simulink model "T6_changeloadmodeltocurrentload_v1"  (R2022b)
settings: Solver=FixedStepAuto  StartTime=0.0  StopTime=48*4  FixedStep=0.01  RelTol=1e-3
undefined symbols (not defined in the file): cableLV, cableMV, High, Low, LV, MV, Scaling_factor, Ts
libraries: fl_lib x149, nesl_utility x73, simulink x60, ee_lib x9
(part 3 of 3)

== system T6_changeloadmodeltocurrentload_v1/Line21 ==
  Current Sensor : fl_lib/Electrical/Electrical Sensors/Current Sensor
  PS-Simulink Converter : nesl_utility/PS-Simulink Converter  PhysicalDomain=network_engine_domain  SubClassName=ps_output  LeftPortType=input  RightPortType=output  PseudoPeriodic=off  Frequencies=[]  VectorFormat=inherit  Unit=inherit  AffineConversion=off
  Resistor : fl_lib/Electrical/Electrical Elements/Resistor  R=rho*l/A Ohm  i_specify=off  i_priority=None  i=0 A  i_nominal_specify=off  i_nominal_unit=A  i_nominal_value=1  v_specify=off  v_priority=None  v=0 V  v_nominal_specify=off  v_nominal_unit=V  v_nominal_value=1
  Resistor1 : fl_lib/Electrical/Electrical Elements/Resistor  R=rho*l/A Ohm  i_specify=off  i_priority=None  i=0 A  i_nominal_specify=off  i_nominal_unit=A  i_nominal_value=1  v_specify=off  v_priority=None  v=0 V  v_nominal_specify=off  v_nominal_unit=V  v_nominal_value=1
  Scope : Scope
  Simscape Bus2 : SimscapeBus  HierarchyStrings=High;Low
  Simscape Bus3 : SimscapeBus  HierarchyStrings=High;Low
  In : PMIOPort  Side=Left
  Out : PMIOPort  Port=2  Side=Right
  wires:
  PS-Simulink Converter/1 -> Scope/1
  connections:
  Simscape Bus2/LConn1 -- Resistor/LConn1
  Simscape Bus3/LConn2 -- Resistor1/RConn1
  Simscape Bus2/RConn1 -- In/RConn1
  Resistor1/LConn1 -- Simscape Bus2/LConn2
  Simscape Bus3/RConn1 -- Out/RConn1
  Current Sensor/LConn1 -- Resistor/RConn1
  Current Sensor/RConn2 -- Simscape Bus3/LConn1
  PS-Simulink Converter/LConn1 -- Current Sensor/RConn1

== system T6_changeloadmodeltocurrentload_v1/Line22 ==
  Current Sensor : fl_lib/Electrical/Electrical Sensors/Current Sensor
  PS-Simulink Converter : nesl_utility/PS-Simulink Converter  PhysicalDomain=network_engine_domain  SubClassName=ps_output  LeftPortType=input  RightPortType=output  PseudoPeriodic=off  Frequencies=[]  VectorFormat=inherit  Unit=inherit  AffineConversion=off
  PS-Simulink Converter1 : nesl_utility/PS-Simulink Converter  PhysicalDomain=network_engine_domain  SubClassName=ps_output  LeftPortType=input  RightPortType=output  PseudoPeriodic=off  Frequencies=[]  VectorFormat=inherit  Unit=inherit  AffineConversion=off
  Resistor : fl_lib/Electrical/Electrical Elements/Resistor  R=rho*l/A Ohm  i_specify=off  i_priority=None  i=0 A  i_nominal_specify=off  i_nominal_unit=A  i_nominal_value=1  v_specify=off  v_priority=None  v=0 V  v_nominal_specify=off  v_nominal_unit=V  v_nominal_value=1
  Resistor1 : fl_lib/Electrical/Electrical Elements/Resistor  R=rho*l/A Ohm  i_specify=off  i_priority=None  i=0 A  i_nominal_specify=off  i_nominal_unit=A  i_nominal_value=1  v_specify=off  v_priority=None  v=0 V  v_nominal_specify=off  v_nominal_unit=V  v_nominal_value=1
  Scope : Scope
  Simscape Bus2 : SimscapeBus  HierarchyStrings=High;Low
  Simscape Bus3 : SimscapeBus  HierarchyStrings=High;Low
  Voltage Sensor : fl_lib/Electrical/Electrical Sensors/Voltage Sensor
  In : PMIOPort  Side=Left
  Out : PMIOPort  Port=2  Side=Right
  tag scope: Bus_Current=global, Bus_Voltage=global
  wires:
  PS-Simulink Converter/1 -> [Bus_Voltage]
  PS-Simulink Converter1/1 -> Scope/1, [Bus_Current]
  connections:
  Simscape Bus3/RConn1 -- Out/RConn1
  Resistor1/LConn1 -- Simscape Bus2/LConn2
  Simscape Bus3/LConn1 -- Voltage Sensor/RConn2 -- Resistor/RConn1
  Simscape Bus2/RConn1 -- In/RConn1
  Simscape Bus3/LConn2 -- Resistor1/RConn1
  PS-Simulink Converter/LConn1 -- Voltage Sensor/RConn1
  Current Sensor/RConn2 -- Voltage Sensor/LConn1 -- Resistor/LConn1
  Current Sensor/LConn1 -- Simscape Bus2/LConn1
  PS-Simulink Converter1/LConn1 -- Current Sensor/RConn1

== system T6_changeloadmodeltocurrentload_v1/Line3 ==
  Resistor : fl_lib/Electrical/Electrical Elements/Resistor  R=rho*l/A Ohm  i_specify=off  i_priority=None  i=0 A  i_nominal_specify=off  i_nominal_unit=A  i_nominal_value=1  v_specify=off  v_priority=None  v=0 V  v_nominal_specify=off  v_nominal_unit=V  v_nominal_value=1
  Resistor1 : fl_lib/Electrical/Electrical Elements/Resistor  R=rho*l/A Ohm  i_specify=off  i_priority=None  i=0 A  i_nominal_specify=off  i_nominal_unit=A  i_nominal_value=1  v_specify=off  v_priority=None  v=0 V  v_nominal_specify=off  v_nominal_unit=V  v_nominal_value=1
  Simscape Bus2 : SimscapeBus  HierarchyStrings=High;Low
  Simscape Bus3 : SimscapeBus  HierarchyStrings=High;Low
  In : PMIOPort  Side=Left
  Out : PMIOPort  Port=2  Side=Right
  connections:
  Simscape Bus2/LConn1 -- Resistor/LConn1
  Simscape Bus3/LConn2 -- Resistor1/RConn1
  Simscape Bus2/RConn1 -- In/RConn1
  Simscape Bus3/LConn1 -- Resistor/RConn1
  Resistor1/LConn1 -- Simscape Bus2/LConn2
  Simscape Bus3/RConn1 -- Out/RConn1

== system T6_changeloadmodeltocurrentload_v1/Line4 ==
  Resistor : fl_lib/Electrical/Electrical Elements/Resistor  R=rho*l/A Ohm  i_specify=off  i_priority=None  i=0 A  i_nominal_specify=off  i_nominal_unit=A  i_nominal_value=1  v_specify=off  v_priority=None  v=0 V  v_nominal_specify=off  v_nominal_unit=V  v_nominal_value=1
  Resistor1 : fl_lib/Electrical/Electrical Elements/Resistor  R=rho*l/A Ohm  i_specify=off  i_priority=None  i=0 A  i_nominal_specify=off  i_nominal_unit=A  i_nominal_value=1  v_specify=off  v_priority=None  v=0 V  v_nominal_specify=off  v_nominal_unit=V  v_nominal_value=1
  Simscape Bus2 : SimscapeBus  HierarchyStrings=High;Low
  Simscape Bus3 : SimscapeBus  HierarchyStrings=High;Low
  In : PMIOPort  Side=Left
  Out : PMIOPort  Port=2  Side=Right
  connections:
  Simscape Bus3/RConn1 -- Out/RConn1
  Resistor1/LConn1 -- Simscape Bus2/LConn2
  Simscape Bus3/LConn1 -- Resistor/RConn1
  Simscape Bus2/RConn1 -- In/RConn1
  Simscape Bus3/LConn2 -- Resistor1/RConn1
  Simscape Bus2/LConn1 -- Resistor/LConn1

== system T6_changeloadmodeltocurrentload_v1/Line5 ==
  Resistor : fl_lib/Electrical/Electrical Elements/Resistor  R=rho*l/A Ohm  i_specify=off  i_priority=None  i=0 A  i_nominal_specify=off  i_nominal_unit=A  i_nominal_value=1  v_specify=off  v_priority=None  v=0 V  v_nominal_specify=off  v_nominal_unit=V  v_nominal_value=1
  Resistor1 : fl_lib/Electrical/Electrical Elements/Resistor  R=rho*l/A Ohm  i_specify=off  i_priority=None  i=0 A  i_nominal_specify=off  i_nominal_unit=A  i_nominal_value=1  v_specify=off  v_priority=None  v=0 V  v_nominal_specify=off  v_nominal_unit=V  v_nominal_value=1
  Simscape Bus2 : SimscapeBus  HierarchyStrings=High;Low
  Simscape Bus3 : SimscapeBus  HierarchyStrings=High;Low
  In : PMIOPort  Side=Left
  Out : PMIOPort  Port=2  Side=Right
  connections:
  Simscape Bus2/LConn1 -- Resistor/LConn1
  Simscape Bus3/LConn2 -- Resistor1/RConn1
  Simscape Bus2/RConn1 -- In/RConn1
  Simscape Bus3/LConn1 -- Resistor/RConn1
  Resistor1/LConn1 -- Simscape Bus2/LConn2
  Simscape Bus3/RConn1 -- Out/RConn1

== system T6_changeloadmodeltocurrentload_v1/Line6 ==
  Resistor : fl_lib/Electrical/Electrical Elements/Resistor  R=rho*l/A Ohm  i_specify=off  i_priority=None  i=0 A  i_nominal_specify=off  i_nominal_unit=A  i_nominal_value=1  v_specify=off  v_priority=None  v=0 V  v_nominal_specify=off  v_nominal_unit=V  v_nominal_value=1
  Resistor1 : fl_lib/Electrical/Electrical Elements/Resistor  R=rho*l/A Ohm  i_specify=off  i_priority=None  i=0 A  i_nominal_specify=off  i_nominal_unit=A  i_nominal_value=1  v_specify=off  v_priority=None  v=0 V  v_nominal_specify=off  v_nominal_unit=V  v_nominal_value=1
  Simscape Bus2 : SimscapeBus  HierarchyStrings=High;Low
  Simscape Bus3 : SimscapeBus  HierarchyStrings=High;Low
  In : PMIOPort  Side=Left
  Out : PMIOPort  Port=2  Side=Right
  connections:
  Simscape Bus3/RConn1 -- Out/RConn1
  Resistor1/LConn1 -- Simscape Bus2/LConn2
  Simscape Bus3/LConn1 -- Resistor/RConn1
  Simscape Bus2/RConn1 -- In/RConn1
  Simscape Bus3/LConn2 -- Resistor1/RConn1
  Simscape Bus2/LConn1 -- Resistor/LConn1

== system T6_changeloadmodeltocurrentload_v1/Line7 ==
  Resistor : fl_lib/Electrical/Electrical Elements/Resistor  R=rho*l/A Ohm  i_specify=off  i_priority=None  i=0 A  i_nominal_specify=off  i_nominal_unit=A  i_nominal_value=1  v_specify=off  v_priority=None  v=0 V  v_nominal_specify=off  v_nominal_unit=V  v_nominal_value=1
  Resistor1 : fl_lib/Electrical/Electrical Elements/Resistor  R=rho*l/A Ohm  i_specify=off  i_priority=None  i=0 A  i_nominal_specify=off  i_nominal_unit=A  i_nominal_value=1  v_specify=off  v_priority=None  v=0 V  v_nominal_specify=off  v_nominal_unit=V  v_nominal_value=1
  Simscape Bus2 : SimscapeBus  HierarchyStrings=High;Low
  Simscape Bus3 : SimscapeBus  HierarchyStrings=High;Low
  In : PMIOPort  Side=Left
  Out : PMIOPort  Port=2  Side=Right
  connections:
  Simscape Bus2/LConn1 -- Resistor/LConn1
  Simscape Bus3/LConn2 -- Resistor1/RConn1
  Simscape Bus2/RConn1 -- In/RConn1
  Simscape Bus3/LConn1 -- Resistor/RConn1
  Resistor1/LConn1 -- Simscape Bus2/LConn2
  Simscape Bus3/RConn1 -- Out/RConn1

== system T6_changeloadmodeltocurrentload_v1/Line8 ==
  Current Sensor : fl_lib/Electrical/Electrical Sensors/Current Sensor
  PS-Simulink Converter : nesl_utility/PS-Simulink Converter  PhysicalDomain=network_engine_domain  SubClassName=ps_output  LeftPortType=input  RightPortType=output  PseudoPeriodic=off  Frequencies=[]  VectorFormat=inherit  Unit=inherit  AffineConversion=off
  Resistor : fl_lib/Electrical/Electrical Elements/Resistor  R=rho*l/A Ohm  i_specify=off  i_priority=None  i=0 A  i_nominal_specify=off  i_nominal_unit=A  i_nominal_value=1  v_specify=off  v_priority=None  v=0 V  v_nominal_specify=off  v_nominal_unit=V  v_nominal_value=1
  Resistor1 : fl_lib/Electrical/Electrical Elements/Resistor  R=rho*l/A Ohm  i_specify=off  i_priority=None  i=0 A  i_nominal_specify=off  i_nominal_unit=A  i_nominal_value=1  v_specify=off  v_priority=None  v=0 V  v_nominal_specify=off  v_nominal_unit=V  v_nominal_value=1
  Scope : Scope
  Simscape Bus2 : SimscapeBus  HierarchyStrings=High;Low
  Simscape Bus3 : SimscapeBus  HierarchyStrings=High;Low
  In : PMIOPort  Side=Left
  Out : PMIOPort  Port=2  Side=Right
  wires:
  PS-Simulink Converter/1 -> Scope/1
  connections:
  Simscape Bus2/LConn1 -- Resistor/LConn1
  Simscape Bus3/LConn2 -- Resistor1/RConn1
  Simscape Bus2/RConn1 -- In/RConn1
  Resistor1/LConn1 -- Simscape Bus2/LConn2
  Simscape Bus3/RConn1 -- Out/RConn1
  Resistor/RConn1 -- Current Sensor/LConn1
  Current Sensor/RConn2 -- Simscape Bus3/LConn1
  PS-Simulink Converter/LConn1 -- Current Sensor/RConn1

== system T6_changeloadmodeltocurrentload_v1/Line9 ==
  Resistor : fl_lib/Electrical/Electrical Elements/Resistor  R=rho*l/A Ohm  i_specify=off  i_priority=None  i=0 A  i_nominal_specify=off  i_nominal_unit=A  i_nominal_value=1  v_specify=off  v_priority=None  v=0 V  v_nominal_specify=off  v_nominal_unit=V  v_nominal_value=1
  Resistor1 : fl_lib/Electrical/Electrical Elements/Resistor  R=rho*l/A Ohm  i_specify=off  i_priority=None  i=0 A  i_nominal_specify=off  i_nominal_unit=A  i_nominal_value=1  v_specify=off  v_priority=None  v=0 V  v_nominal_specify=off  v_nominal_unit=V  v_nominal_value=1
  Simscape Bus2 : SimscapeBus  HierarchyStrings=High;Low
  Simscape Bus3 : SimscapeBus  HierarchyStrings=High;Low
  In : PMIOPort  Side=Left
  Out : PMIOPort  Port=2  Side=Right
  connections:
  Simscape Bus3/RConn1 -- Out/RConn1
  Resistor1/LConn1 -- Simscape Bus2/LConn2
  Simscape Bus3/LConn1 -- Resistor/RConn1
  Simscape Bus2/RConn1 -- In/RConn1
  Simscape Bus3/LConn2 -- Resistor1/RConn1
  Simscape Bus2/LConn1 -- Resistor/LConn1

== system T6_changeloadmodeltocurrentload_v1/Solar power ==
  note: -9
  note: -4
  note: Ns series panel
  Irradiance2 : Inport
  Buck/Boost Converter : Subsystem
      settings: PortSchema="{\"entries\":[{\"content\":{\"sides\":[{\"content\":{\"connectorIds\":[\"LConn1\",\"LConn2\"]},\"type\":\"ConnectorPlacement.EquallySpacedRectSide\",\"uuid\":\"5c021c6f-6d43-4834-8d7d-5513bb4d55a2\"},{\"content\":{\"connectorIds\":[\"RConn1\",\"RConn2\"],\"side\":\"RIGHT\"},\"type\":\"ConnectorPlacement.EquallySpacedRectSide\",\"uuid\":\"9a583822-2cc1-49ae-b5aa-706b08d37e90\"},{\"content\":{\"connectorIds\":[\"In1\"],\"side\":\"TOP\"},\"type\":\"ConnectorPlacement.EquallySpacedRectSide\",\"uuid\":\"d4d092e8-f797-44a8-a681-f8c20d4ba78f\"}]},\"type\":\"ConnectorPlacement.EquallySpacedConnector\",\"uuid\":\"2126b667-6bdd-4954-a062-f2cc2f0ec1c9\"}],\"packageUris\":[\"http://schema.mathworks.com/mf0/Connector/R2020b\"],\"version\":\"1.0\"}"
  Current Sensor2 : fl_lib/Electrical/Electrical Sensors/Current Sensor
  Current-Controlled Current Source : fl_lib/Electrical/Electrical Sources/Current-Controlled Current Source  K=-1*(1-1)  i1_specify=off  i1_priority=None  i1=0 A  i1_nominal_specify=off  i1_nominal_unit=A  i1_nominal_value=1  i2_specify=off  i2_priority=None  i2=0 A  i2_nominal_specify=off  i2_nominal_unit=A  i2_nominal_value=1
      settings: InternalSimscapePortConfiguration="{\"Bottom\":[],\"Left\":[{\"id\":\"p1\",\"label\":\"+\",\"type\":\"foundation.electrical.electrical\"},{\"id\":\"head\",\"label\":\"\",\"type\":\"foundation.electrical.electrical\"}],\"Right\":[{\"id\":\"n1\",\"label\":\"-\",\"type\":\"foundation.electrical.electrical\"},{\"id\":\"tail\",\"label\":\"\",\"type\":\"foundation.electrical.electrical\"}],\"Top\":[]}"
  Current-Controlled Current Source- Scale panel current to Np parallel strings : fl_lib/Electrical/Electrical Sources/Current-Controlled Current Source  K=-1*(1-1)  i1_specify=off  i1_priority=None  i1=0 A  i1_nominal_specify=off  i1_nominal_unit=A  i1_nominal_value=1  i2_specify=off  i2_priority=None  i2=0 A  i2_nominal_specify=off  i2_nominal_unit=A  i2_nominal_value=1
      settings: InternalSimscapePortConfiguration="{\"Bottom\":[],\"Left\":[{\"id\":\"p1\",\"label\":\"+\",\"type\":\"foundation.electrical.electrical\"},{\"id\":\"head\",\"label\":\"\",\"type\":\"foundation.electrical.electrical\"}],\"Right\":[{\"id\":\"n1\",\"label\":\"-\",\"type\":\"foundation.electrical.electrical\"},{\"id\":\"tail\",\"label\":\"\",\"type\":\"foundation.electrical.electrical\"}],\"Top\":[]}"
  ERef : fl_lib/Electrical/Electrical Elements/Electrical Reference
  MPPT : Subsystem
  PS-Simulink Converter1 : nesl_utility/PS-Simulink Converter  PhysicalDomain=network_engine_domain  SubClassName=ps_output  LeftPortType=input  RightPortType=output  PseudoPeriodic=off  Frequencies=[]  VectorFormat=1-D array  Unit=inherit  AffineConversion=off
  PS-Simulink Converter4 : nesl_utility/PS-Simulink Converter  PhysicalDomain=network_engine_domain  SubClassName=ps_output  LeftPortType=input  RightPortType=output  PseudoPeriodic=off  Frequencies=[]  VectorFormat=1-D array  Unit=inherit  AffineConversion=off
  Product3 : Product
  Scope : Scope
  Sensing Current : Subsystem
      settings: PortSchema="{\"entries\":[{\"content\":{\"sides\":[{\"content\":{\"connectorIds\":[\"LConn1\"]},\"type\":\"ConnectorPlacement.EquallySpacedRectSide\",\"uuid\":\"08eaf192-3836-4d70-9f6a-c3aee0977ea6\"},{\"content\":{\"connectorIds\":[\"RConn1\"],\"side\":\"RIGHT\"},\"type\":\"ConnectorPlacement.EquallySpacedRectSide\",\"uuid\":\"69615d36-c1bf-4d31-b3e4-77c73286e7c7\"},{\"content\":{\"connectorIds\":[\"Out1\"],\"side\":\"TOP\"},\"type\":\"ConnectorPlacement.EquallySpacedRectSide\",\"uuid\":\"21e31d90-f675-47e5-98f5-1bf7e6a5fdbe\"}]},\"type\":\"ConnectorPlacement.EquallySpacedConnector\",\"uuid\":\"068abd2e-abc9-41d7-b40e-d83d3e3b9346\"}],\"packageUris\":[\"http://schema.mathworks.com/mf0/Connector/R2020b\"],\"version\":\"1.0\"}"
      mask Display: disp('i')
  Simscape Bus1 : SimscapeBus  HierarchyStrings=High;Low
  Simulink-PS Converter2 : nesl_utility/Simulink-PS Converter  PhysicalDomain=network_engine_domain  SubClassName=ps_input  LeftPortType=input  RightPortType=output  PseudoPeriodic=off  Frequencies=[]  NoiseDistribution=none  NoiseParameters=[]  Unit=1  AffineConversion=off  FilteringAndDerivatives=provide  SimscapeFilterOrder=1  InputFilterTimeConstant=0.001  UdotUserProvided=0
  Solar Cell1 : ee_lib/Sources/Solar Cell  Tag={'toolbox/physmod/elec/library/m/ee_lib_parts';'Sources/Solar_Cell/Amerisolar/AS_6M30_HC_320W.xml'}  prm=1  Isc=10.00 A  Voc=0.673 V  Is=3.24823447983853e-07 A  Is2=9.37081970792037e-10 A  Iph=10.140005507508 A  Ir0=1000 W/m^2  ec=1.5  N2=2.60259908345858  Rs=0 Ohm  Rp=682.95993142779 Ohm  N_series=60  N_parallel=1  TIPH1=0.000499942933005141 1/K  EG=1.12 eV  TXIS1=4.23641510120988  TXIS2=16.2689137700667  TRS1=0.243341028305912  TRP1=0 % Parameter not set  Tmeas=25 degC  TFIXED=25 degC  thermal_mass=100 % Parameter not set J/K  initial_temperature=25 degC
      settings: AttributesFormatString=Amerisolar:AS_6M30_HC_320W
  Voltage Sensor2 : fl_lib/Electrical/Electrical Sensors/Voltage Sensor
  Voltage-Controlled Voltage Source - Scale panel voltage to Ns series panel : fl_lib/Electrical/Electrical Sources/Voltage-Controlled Voltage Source  K=-1*(21-1)  v1_specify=off  v1_priority=None  v1=0 V  v1_nominal_specify=off  v1_nominal_unit=V  v1_nominal_value=1  v2_specify=off  v2_priority=None  v2=0 V  v2_nominal_specify=off  v2_nominal_unit=V  v2_nominal_value=1
      settings: InternalSimscapePortConfiguration="{\"Bottom\":[],\"Left\":[{\"id\":\"p1\",\"label\":\"+\",\"type\":\"foundation.electrical.electrical\"},{\"id\":\"p2\",\"label\":\"+\",\"type\":\"foundation.electrical.electrical\"}],\"Right\":[{\"id\":\"n1\",\"label\":\"-\",\"type\":\"foundation.electrical.electrical\"},{\"id\":\"n2\",\"label\":\"-\",\"type\":\"foundation.electrical.electrical\"}],\"Top\":[]}"
  sensing voltage : Subsystem
      settings: PortSchema="{\"entries\":[{\"content\":{\"sides\":[{\"content\":{\"connectorIds\":[\"LConn1\"]},\"type\":\"ConnectorPlacement.EquallySpacedRectSide\",\"uuid\":\"08eaf192-3836-4d70-9f6a-c3aee0977ea6\"},{\"content\":{\"connectorIds\":[\"RConn1\"],\"side\":\"RIGHT\"},\"type\":\"ConnectorPlacement.EquallySpacedRectSide\",\"uuid\":\"69615d36-c1bf-4d31-b3e4-77c73286e7c7\"},{\"content\":{\"connectorIds\":[],\"side\":\"TOP\"},\"type\":\"ConnectorPlacement.EquallySpacedRectSide\",\"uuid\":\"21e31d90-f675-47e5-98f5-1bf7e6a5fdbe\"},{\"content\":{\"connectorIds\":[\"Out1\"],\"side\":\"BOTTOM\"},\"type\":\"ConnectorPlacement.EquallySpacedRectSide\",\"uuid\":\"23a77980-6beb-4147-b48e-adf9e1983263\"}]},\"type\":\"ConnectorPlacement.EquallySpacedConnector\",\"uuid\":\"068abd2e-abc9-41d7-b40e-d83d3e3b9346\"}],\"packageUris\":[\"http://schema.mathworks.com/mf0/Connector/R2020b\"],\"version\":\"1.0\"}"
      mask Display: disp('v')
  solaroutput2 : PMIOPort  Side=Left
  tag scope: MPPT_duty_cycle=global, P_PV=global, V_PV=global, V_PV_load=global
  wires:
  MPPT/1(duty_cycle) -> [MPPT_duty_cycle], Buck/Boost Converter/1(duty_cycle)  "duty_cycle"
  PS-Simulink Converter4/1 -> [V_PV_load], Product3/2  "V_PV_load"
  Sensing Current/1(I) -> MPPT/1(I)
  Irradiance2/1 -> Simulink-PS Converter2/1
  sensing voltage/1(V) -> [V_PV], MPPT/2(V)  "V_cell"
  PS-Simulink Converter1/1 -> Scope/1, Product3/1  "I_PV_load"
  Product3/1 -> [P_PV]  "P_PV"
  connections:
  sensing voltage/RConn1 -- ERef/LConn1 -- Current-Controlled Current Source- Scale panel current to Np parallel strings/LConn2 -- Voltage-Controlled Voltage Source - Scale panel voltage to Ns series panel/LConn1 -- Current-Controlled Current Source/LConn2 -- Solar Cell1/RConn1 -- Buck/Boost Converter/LConn2
  Voltage Sensor2/LConn1 -- Current Sensor2/RConn2 -- Simscape Bus1/LConn1
  Voltage-Controlled Voltage Source - Scale panel voltage to Ns series panel/RConn2 -- Voltage-Controlled Voltage Source - Scale panel voltage to Ns series panel/RConn1 -- Current-Controlled Current Source/RConn1 -- Current-Controlled Current Source/RConn2
  Voltage Sensor2/RConn2 -- Simscape Bus1/LConn2 -- Buck/Boost Converter/RConn2
  Sensing Current/LConn1 -- Current-Controlled Current Source- Scale panel current to Np parallel strings/RConn2 -- Current-Controlled Current Source- Scale panel current to Np parallel strings/RConn1
  Sensing Current/RConn1 -- Buck/Boost Converter/LConn1 -- sensing voltage/LConn1
  solaroutput2/RConn1 -- Simscape Bus1/RConn1
  Solar Cell1/LConn2 -- Current-Controlled Current Source/LConn1
  Buck/Boost Converter/RConn1 -- Current Sensor2/LConn1
  PS-Simulink Converter4/LConn1 -- Voltage Sensor2/RConn1
  Simulink-PS Converter2/RConn1 -- Solar Cell1/LConn1
  Current-Controlled Current Source- Scale panel current to Np parallel strings/LConn1 -- Voltage-Controlled Voltage Source - Scale panel voltage to Ns series panel/LConn2
  PS-Simulink Converter1/LConn1 -- Current Sensor2/RConn1

== system T6_changeloadmodeltocurrentload_v1/Subsystem ==
  "  " : simulink/Sources/Repeating Sequence Interpolated  OutValues=|  TimeValues=Allday_timevector  LookUpMeth=Interpolation-Use End Values  tsamp=0.01  OutMin=[]  OutMax=[]  OutDataTypeStr=double  OutputDataTypeScalingMode=double  OutDataType=fixdt(0,8)  OutScaling=2^-10
      | [2.38
      | 2.43
      | 2.50
      | 2.50
      | 2.45
      | 2.30
      | 2.12
      | 2.15
      | 2.03
      | 2.55
      | 2.97
      | 3.30
      | 3.58
      | 3.83
      | 2.98
      | 2.62
      | 2.53
      | 2.35
      | 2.00
      | 1.72
      | 1.90
      | 2.24
      | 2.15
      | 1.99
      | 1.73
      | 1.40
      | 1.27
      | 1.20
      | 1.43
      | 1.74
      | 1.62
      | 1.35
      | 1.21
      | 1.20
      | 0.98
      | 1.41
      | 1.20
      | 2.08
      | 2.65
      | 2.90
      | 3.03
      | 2.47
      | 2.33
      | 1.97
      | 2.38
      | 3.00
      | 3.01
      | 3.75
      | ]
  "  1" : simulink/Sources/Repeating Sequence Interpolated  OutValues=|  TimeValues=Allday_timevector  LookUpMeth=Interpolation-Use End Values  tsamp=0.01  OutMin=[]  OutMax=[]  OutDataTypeStr=double  OutputDataTypeScalingMode=double  OutDataType=fixdt(0,8)  OutScaling=2^-10
      | [1.52
      | 2.00
      | 2.25
      | 2.19
      | 1.97
      | 1.88
      | 1.99
      | 2.20
      | 2.13
      | 2.47
      | 2.68
      | 2.41
      | 2.85
      | 3.00
      | 3.11
      | 3.38
      | 3.38
      | 3.22
      | 2.93
      | 2.41
      | 1.90
      | 1.46
      | 1.63
      | 1.93
      | 1.93
      | 1.82
      | 1.72
      | 1.76
      | 1.87
      | 2.03
      | 2.21
      | 2.43
      | 2.53
      | 2.73
      | 3.07
      | 2.98
      | 3.38
      | 3.42
      | 3.41
      | 3.57
      | 3.61
      | 3.13
      | 2.60
      | 2.20
      | 1.94
      | 1.79
      | 2.28
      | 2.72
      | ]
  "  2" : simulink/Sources/Repeating Sequence Interpolated  OutValues=|  TimeValues=Allday_timevector  LookUpMeth=Interpolation-Use End Values  tsamp=0.01  OutMin=[]  OutMax=[]  OutDataTypeStr=double  OutputDataTypeScalingMode=double  OutDataType=fixdt(0,8)  OutScaling=2^-10
      | [3.40
      | 3.35
      | 3.12
      | 2.74
      | 2.37
      | 2.18
      | 2.30
      | 2.50
      | 2.53
      | 2.74
      | 3.08
      | 3.20
      | 3.11
      | 3.13
      | 3.00
      | 2.60
      | 2.50
      | 2.49
      | 1.93
      | 1.87
      | 1.77
      | 1.89
      | 2.14
      | 2.40
      | 2.23
      | 1.84
      | 1.44
      | 1.22
      | 1.18
      | 1.58
      | 2.32
      | 2.86
      | 2.93
      | 2.75
      | 2.68
      | 3.38
      | 3.88
      | 3.13
      | 2.95
      | 2.68
      | 2.50
      | 2.18
      | 1.75
      | 1.70
      | 1.41
      | 1.45
      | 1.40
      | 1.57
      | ]
  "  3" : simulink/Sources/Repeating Sequence Interpolated  OutValues=|  TimeValues=Allday_timevector  LookUpMeth=Interpolation-Use End Values  tsamp=0.01  OutMin=[]  OutMax=[]  OutDataTypeStr=double  OutputDataTypeScalingMode=double  OutDataType=fixdt(0,8)  OutScaling=2^-10
      | [6.20
      | 6.47
      | 6.65
      | 6.70
      | 6.67
      | 6.51
      | 6.27
      | 6.12
      | 5.23
      | 4.95
      | 5.80
      | 6.35
      | 6.57
      | 6.13
      | 6.18
      | 6.83
      | 6.19
      | 6.07
      | 5.72
      | 5.20
      | 4.67
      | 4.67
      | 4.80
      | 5.17
      | 5.25
      | 5.36
      | 5.13
      | 4.83
      | 4.62
      | 4.74
      | 4.95
      | 4.72
      | 4.23
      | 4.55
      | 4.95
      | 5.37
      | 5.82
      | 5.82
      | 5.15
      | 4.62
      | 4.33
      | 3.82
      | 3.49
      | 3.46
      | 2.80
      | 2.87
      | 2.88
      | 2.89
      | ]
  MATLAB Function : MATLAB Function  TreatAsAtomicUnit=on
  wind : Outport
  wires:
  [Button1selected] -> MATLAB Function/1(button1)
  "  2"/1 -> MATLAB Function/7(data3)
  [Button3selected] -> MATLAB Function/3(button3)
  [Button4selected] -> MATLAB Function/4(button4)
  [Button2selected] -> MATLAB Function/2(button2)
  "  "/1 -> MATLAB Function/5(data1)
  MATLAB Function/1(y) -> wind/1
  "  1"/1 -> MATLAB Function/6(data2)
  "  3"/1 -> MATLAB Function/8(data4)

== system T6_changeloadmodeltocurrentload_v1/Subsystem1 ==
  "  " : simulink/Sources/Repeating Sequence Interpolated  OutValues=|  TimeValues=Allday_timevector  LookUpMeth=Interpolation-Use End Values  tsamp=0.01  OutMin=[]  OutMax=[]  OutDataTypeStr=double  OutputDataTypeScalingMode=double  OutDataType=fixdt(0,8)  OutScaling=2^-10
      | [0.00
      | 0.00
      | 0.00
      | 0.00
      | 0.00
      | 0.00
      | 6.25
      | 147.50
      | 298.75
      | 185.42
      | 130.83
      | 144.58
      | 146.67
      | 150.00
      | 204.17
      | 394.58
      | 154.17
      | 50.83
      | 11.67
      | 0.00
      | 0.00
      | 0.00
      | 0.00
      | 0.00
      | 0.00
      | 0.00
      | 0.00
      | 0.00
      | 0.00
      | 0.00
      | 3.75
      | 74.17
      | 298.33
      | 467.50
      | 486.25
      | 667.92
      | 716.25
      | 464.17
      | 315.83
      | 259.17
      | 292.08
      | 245.00
      | 67.92
      | 0.00
      | 0.00
      | 0.00
      | 0.00
      | 0.00
      | ]
  "  1" : simulink/Sources/Repeating Sequence Interpolated  OutValues=|  TimeValues=Allday_timevector  LookUpMeth=Interpolation-Use End Values  tsamp=0.01  OutMin=[]  OutMax=[]  OutDataTypeStr=double  OutputDataTypeScalingMode=double  OutDataType=fixdt(0,8)  OutScaling=2^-10
      | [0.00
      | 0.00
      | 0.00
      | 0.00
      | 0.00
      | 7.08
      | 36.67
      | 183.75
      | 364.17
      | 364.17
      | 436.25
      | 618.33
      | 503.33
      | 567.08
      | 691.67
      | 644.17
      | 580.83
      | 506.25
      | 501.25
      | 370.83
      | 212.92
      | 56.25
      | 0.00
      | 0.00
      | 0.00
      | 0.00
      | 0.00
      | 0.00
      | 0.00
      | 28.75
      | 160.83
      | 321.25
      | 462.50
      | 519.58
      | 562.08
      | 654.17
      | 777.50
      | 950.83
      | 946.67
      | 895.83
      | 704.17
      | 580.83
      | 432.92
      | 248.33
      | 120.83
      | 16.67
      | 0.00
      | 0.00
      | ]
  "  2" : simulink/Sources/Repeating Sequence Interpolated  OutValues=|  TimeValues=Allday_timevector  LookUpMeth=Interpolation-Use End Values  tsamp=0.01  OutMin=[]  OutMax=[]  OutDataTypeStr=double  OutputDataTypeScalingMode=double  OutDataType=fixdt(0,8)  OutScaling=2^-10
      | [0.00
      | 0.00
      | 0.00
      | 0.00
      | 0.00
      | 0.00
      | 0.00
      | 30.42
      | 189.17
      | 357.50
      | 501.25
      | 612.92
      | 680.00
      | 706.67
      | 605.00
      | 356.25
      | 303.75
      | 325.83
      | 180.83
      | 25.00
      | 0.00
      | 0.00
      | 0.00
      | 0.00
      | 0.00
      | 0.00
      | 0.00
      | 0.00
      | 0.00
      | 0.00
      | 0.00
      | 5.83
      | 36.67
      | 69.58
      | 100.42
      | 121.67
      | 135.42
      | 140.00
      | 134.17
      | 121.25
      | 99.58
      | 69.58
      | 34.58
      | 4.17
      | 0.00
      | 0.00
      | 0.00
      | 0.00
      | ]
  "  3" : simulink/Sources/Repeating Sequence Interpolated  OutValues=|  TimeValues=Allday_timevector  LookUpMeth=Interpolation-Use End Values  tsamp=0.01  OutMin=[]  OutMax=[]  OutDataTypeStr=double  OutputDataTypeScalingMode=double  OutDataType=fixdt(0,8)  OutScaling=2^-10
      | [0.00
      | 0.00
      | 0.00
      | 0.00
      | 0.00
      | 0.00
      | 0.00
      | 0.00
      | 7.08
      | 40.83
      | 72.50
      | 69.17
      | 70.00
      | 65.00
      | 51.67
      | 31.67
      | 5.00
      | 0.00
      | 0.00
      | 0.00
      | 0.00
      | 0.00
      | 0.00
      | 0.00
      | 0.00
      | 0.00
      | 0.00
      | 0.00
      | 0.00
      | 0.00
      | 0.00
      | 0.00
      | 17.92
      | 79.17
      | 133.33
      | 212.50
      | 147.50
      | 118.33
      | 98.33
      | 68.75
      | 10.83
      | 0.00
      | 0.00
      | 0.00
      | 0.00
      | 0.00
      | 0.00
      | 0.00
      | ]
  MATLAB Function : MATLAB Function  TreatAsAtomicUnit=on
  irradiance : Outport
  wires:
  MATLAB Function/1(y) -> irradiance/1
  "  "/1 -> MATLAB Function/5(data1)
  [Button2selected] -> MATLAB Function/2(button2)
  [Button4selected] -> MATLAB Function/4(button4)
  [Button3selected] -> MATLAB Function/3(button3)
  "  2"/1 -> MATLAB Function/7(data3)
  [Button1selected] -> MATLAB Function/1(button1)
  "  1"/1 -> MATLAB Function/6(data2)
  "  3"/1 -> MATLAB Function/8(data4)

== system T6_changeloadmodeltocurrentload_v1/Subsystem10 ==
  Resistor : fl_lib/Electrical/Electrical Elements/Resistor  R=rho*l/A Ohm  i_specify=off  i_priority=None  i=0 A  i_nominal_specify=off  i_nominal_unit=A  i_nominal_value=1  v_specify=off  v_priority=None  v=0 V  v_nominal_specify=off  v_nominal_unit=V  v_nominal_value=1
  Resistor1 : fl_lib/Electrical/Electrical Elements/Resistor  R=rho*l/A Ohm  i_specify=off  i_priority=None  i=0 A  i_nominal_specify=off  i_nominal_unit=A  i_nominal_value=1  v_specify=off  v_priority=None  v=0 V  v_nominal_specify=off  v_nominal_unit=V  v_nominal_value=1
  Simscape Bus2 : SimscapeBus  HierarchyStrings=High;Low
  Simscape Bus3 : SimscapeBus  HierarchyStrings=High;Low
  In : PMIOPort  Side=Left
  Out : PMIOPort  Port=2  Side=Right
  connections:
  Simscape Bus3/RConn1 -- Out/RConn1
  Resistor1/LConn1 -- Simscape Bus2/LConn2
  Simscape Bus3/LConn1 -- Resistor/RConn1
  Simscape Bus2/RConn1 -- In/RConn1
  Simscape Bus3/LConn2 -- Resistor1/RConn1
  Simscape Bus2/LConn1 -- Resistor/LConn1

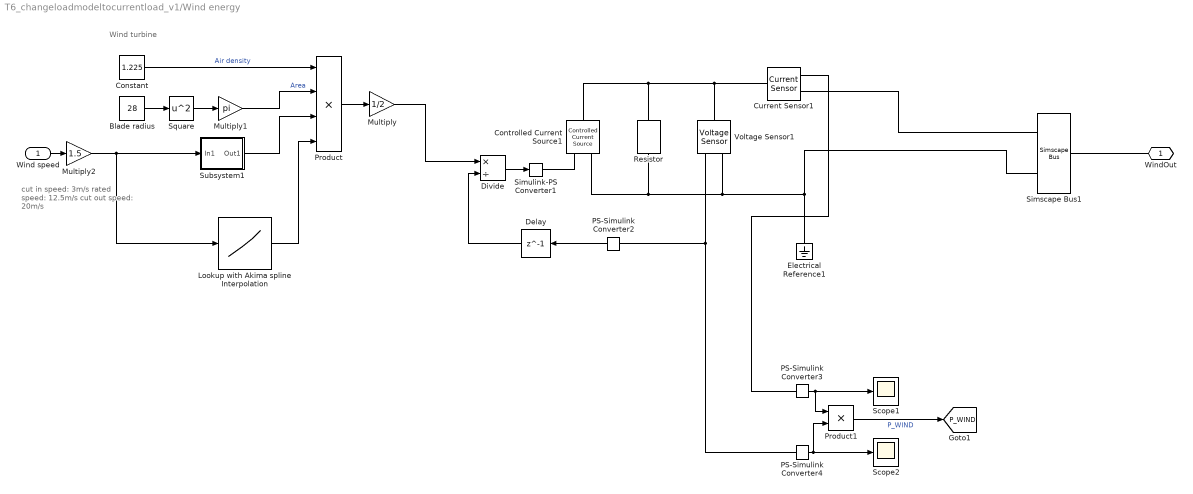
== system T6_changeloadmodeltocurrentload_v1/Wind energy ==
  note: cut in speed: 3m/s
      | rated speed: 12.5m/s
      | cut out speed: 20m/s
  note: Wind turbine
  Wind speed : Inport
  Blade radius : Constant  Value=28
  Constant : Constant  Value=1.225
  Controlled Current Source1 : fl_lib/Electrical/Electrical Sources/Controlled Current Source
  Current Sensor1 : fl_lib/Electrical/Electrical Sensors/Current Sensor
  Delay : Delay  DelayLength=1  InitialCondition=MV
  Divide : Product  Inputs=*/
  Electrical Reference1 : fl_lib/Electrical/Electrical Elements/Electrical Reference
  Lookup with Akima spline Interpolation : Lookup_n-D  NumberOfTableDimensions=1  BreakpointsForDimension1=[0;1;2;3;4;5;6;7;8;9;10;11;12;13;14;15;16;17;18;19;20;21;22;23;24;25;26;27;28]  Table=[0;0;0;0.228;0.322;0.38;0.408;0.413;0.418;0.419;0.419;0.401;0.378;0.305;0.244;0.199;0.164;0.136;0.115;0.098;0.084;0.072;0.063;0.055;0.048;0.042;0;0;0]  InterpMethod=Akima spline  InternalRulePriority=Speed  OutDataTypeStr=double  RndMeth=Simplest
  Multiply : Gain  Gain=1/2
  Multiply1 : Gain  Gain=pi
  Multiply2 : Gain  Gain=1.5
  PS-Simulink Converter2 : nesl_utility/PS-Simulink Converter  PhysicalDomain=network_engine_domain  SubClassName=ps_output  LeftPortType=input  RightPortType=output  PseudoPeriodic=off  Frequencies=[]  VectorFormat=inherit  Unit=inherit  AffineConversion=off
  PS-Simulink Converter3 : nesl_utility/PS-Simulink Converter  PhysicalDomain=network_engine_domain  SubClassName=ps_output  LeftPortType=input  RightPortType=output  PseudoPeriodic=off  Frequencies=[]  VectorFormat=inherit  Unit=inherit  AffineConversion=off
  PS-Simulink Converter4 : nesl_utility/PS-Simulink Converter  PhysicalDomain=network_engine_domain  SubClassName=ps_output  LeftPortType=input  RightPortType=output  PseudoPeriodic=off  Frequencies=[]  VectorFormat=inherit  Unit=inherit  AffineConversion=off
  Product : Product  Inputs=4
  Product1 : Product
  Resistor : fl_lib/Electrical/Electrical Elements/Resistor  R=1e9 Ohm  i_specify=off  i_priority=None  i=0 A  i_nominal_specify=off  i_nominal_unit=A  i_nominal_value=1  v_specify=off  v_priority=None  v=0 V  v_nominal_specify=off  v_nominal_unit=V  v_nominal_value=1
  Scope1 : Scope
  Scope2 : Scope
  Simscape Bus1 : SimscapeBus  HierarchyStrings=High;Low
  Simulink-PS Converter1 : nesl_utility/Simulink-PS Converter  PhysicalDomain=network_engine_domain  SubClassName=ps_input  LeftPortType=input  RightPortType=output  PseudoPeriodic=off  Frequencies=[]  NoiseDistribution=none  NoiseParameters=[]  Unit=1  AffineConversion=off  FilteringAndDerivatives=provide  SimscapeFilterOrder=1  InputFilterTimeConstant=0.001  UdotUserProvided=0
  Square : Math  Operator=square
  Subsystem1 : Subsystem
      mask Display: disp('Vw^3');
  Voltage Sensor1 : fl_lib/Electrical/Electrical Sensors/Voltage Sensor
  WindOut : PMIOPort  Side=Right
  tag scope: P_WIND=global
  wires:
  Lookup with Akima spline Interpolation/1 -> Product/4
  Multiply1/1 -> Product/2  "Area"
  Blade radius/1 -> Square/1
  Square/1 -> Multiply1/1
  Constant/1 -> Product/1  "Air density"
  Wind speed/1 -> Multiply2/1
  Product/1 -> Multiply/1
  Subsystem1/1(Out1) -> Product/3
  Delay/1 -> Divide/2
  PS-Simulink Converter4/1 -> Product1/2, Scope2/1
  Divide/1 -> Simulink-PS Converter1/1
  PS-Simulink Converter3/1 -> Product1/1, Scope1/1
  Product1/1 -> [P_WIND]  "P_WIND"
  Multiply/1 -> Divide/1
  PS-Simulink Converter2/1 -> Delay/1
  Multiply2/1 -> Lookup with Akima spline Interpolation/1, Subsystem1/1(In1)
  connections:
  WindOut/RConn1 -- Simscape Bus1/RConn1
  Controlled Current Source1/RConn2 -- Voltage Sensor1/RConn2 -- Simscape Bus1/LConn2 -- Electrical Reference1/LConn1 -- Resistor/RConn1
  Resistor/LConn1 -- Current Sensor1/LConn1 -- Voltage Sensor1/LConn1 -- Controlled Current Source1/LConn1
  PS-Simulink Converter4/LConn1 -- Voltage Sensor1/RConn1 -- PS-Simulink Converter2/LConn1
  PS-Simulink Converter3/LConn1 -- Current Sensor1/RConn1
  Simulink-PS Converter1/RConn1 -- Controlled Current Source1/RConn1
  Simscape Bus1/LConn1 -- Current Sensor1/RConn2

== system T6_changeloadmodeltocurrentload_v1/Solar power/Buck//Boost Converter ==
  duty_cycle : Inport
  Average-Value DC-DC Converter : ee_lib/Semiconductors & Converters/Converters/Average-Value DC-DC Converter  control_option=ee.enum.converters.controlinput.dutycycle  converter_type=ee.enum.converters.dcdctype.buckboost  efficiency_option=ee.enum.converters.efficiency.constant  efficiency_fixed=100  i_vec=[0, 2, 5] A  efficiency_vec=[90, 95, 98]
      settings: InternalSimscapePortConfiguration="{\"Bottom\":[],\"Left\":[{\"id\":\"DutyCycle\",\"label\":\"DutyCycle\",\"type\":\"input\"},{\"id\":\"p1\",\"label\":\"1+\",\"type\":\"foundation.electrical.electrical\"},{\"id\":\"n1\",\"label\":\"1-\",\"type\":\"foundation.electrical.electrical\"}],\"Right\":[{\"id\":\"p2\",\"label\":\"2+\",\"type\":\"foundation.electrical.electrical\"},{\"id\":\"n2\",\"label\":\"2-\",\"type\":\"foundation.electrical.electrical\"}],\"Top\":[]}"
  Simulink-PS Converter : nesl_utility/Simulink-PS Converter  PhysicalDomain=network_engine_domain  SubClassName=ps_input  LeftPortType=input  RightPortType=output  PseudoPeriodic=off  Frequencies=[]  NoiseDistribution=none  NoiseParameters=[]  Unit=1  AffineConversion=off  FilteringAndDerivatives=provide  SimscapeFilterOrder=1  InputFilterTimeConstant=0.001  UdotUserProvided=0
  Unit Delay : UnitDelay  InitialCondition=0.8  SampleTime=-1  HasFrameUpgradeWarning=on
  +s : PMIOPort  Side=Left
  -s : PMIOPort  Port=2  Side=Left
  -l : PMIOPort  Port=3  Side=Right
  +l : PMIOPort  Port=4  Side=Right
  wires:
  Unit Delay/1 -> Simulink-PS Converter/1
  duty_cycle/1 -> Unit Delay/1
  connections:
  Average-Value DC-DC Converter/RConn1 -- -l/RConn1
  +l/RConn1 -- Average-Value DC-DC Converter/RConn2
  Simulink-PS Converter/RConn1 -- Average-Value DC-DC Converter/LConn1
  Average-Value DC-DC Converter/LConn3 -- -s/RConn1
  +s/RConn1 -- Average-Value DC-DC Converter/LConn2

== system T6_changeloadmodeltocurrentload_v1/Solar power/MPPT ==
  note: Initial value for D output (Dinit)
  note: Increment value used to increase/decrease (DeltaD)
  note: Upper limit for D (Dmax)
  note: Lower limit for D (Dmin)
  I : Inport
  V : Inport  Port=2
  Enable MPPT : Step  Time=0.1  SampleTime=0.01
  Iph_ : Constant  Value=0.8
  Iph_1 : Constant  Value=0.85
  Iph_2 : Constant  Value=0.1
  Iph_3 : Constant  Value=3e-3*0.5
  "MPPT Controller using Perturb & Observe technique " : MATLAB Function  SystemSampleTime=Ts
  Mux : Mux
  Unit Delay : UnitDelay  InitialCondition=0.6  SampleTime=-1  HasFrameUpgradeWarning=on
  duty_cycle : Outport
  wires:
  V/1 -> "MPPT Controller using Perturb & Observe technique "/3(V)
  Mux/1 -> "MPPT Controller using Perturb & Observe technique "/1(Param)
  Iph_1/1 -> Mux/2
  Iph_/1 -> Mux/1
  Iph_2/1 -> Mux/3
  "MPPT Controller using Perturb & Observe technique "/1(D) -> Unit Delay/1  "duty_cycle"
  Iph_3/1 -> Mux/4
  Enable MPPT/1 -> "MPPT Controller using Perturb & Observe technique "/2(Enabled)
  I/1 -> "MPPT Controller using Perturb & Observe technique "/4(I)
  Unit Delay/1 -> duty_cycle/1

== system T6_changeloadmodeltocurrentload_v1/Solar power/Sensing Current ==
  Current Sensor : fl_lib/Electrical/Electrical Sensors/Current Sensor
  PS-Simulink/I : nesl_utility/PS-Simulink Converter  PhysicalDomain=network_engine_domain  SubClassName=ps_output  LeftPortType=input  RightPortType=output  PseudoPeriodic=off  Frequencies=[]  VectorFormat=1-D array  Unit=1  AffineConversion=off
  + : PMIOPort  Side=Left
  - : PMIOPort  Port=2  Side=Right
  I : Outport
  wires:
  PS-Simulink/I/1 -> I/1
  connections:
  -/RConn1 -- Current Sensor/RConn2
  Current Sensor/LConn1 -- +/RConn1
  Current Sensor/RConn1 -- PS-Simulink/I/LConn1

== system T6_changeloadmodeltocurrentload_v1/Solar power/sensing voltage ==
  PS-Simulink Converter : nesl_utility/PS-Simulink Converter  PhysicalDomain=network_engine_domain  SubClassName=ps_output  LeftPortType=input  RightPortType=output  PseudoPeriodic=off  Frequencies=[]  VectorFormat=1-D array  Unit=inherit  AffineConversion=off
  Voltage Sensor : fl_lib/Electrical/Electrical Sensors/Voltage Sensor
  + : PMIOPort  Side=Left
  - : PMIOPort  Port=2  Side=Right
  V : Outport
  wires:
  PS-Simulink Converter/1 -> V/1
  connections:
  Voltage Sensor/LConn1 -- +/RConn1
  Voltage Sensor/RConn2 -- -/RConn1
  Voltage Sensor/RConn1 -- PS-Simulink Converter/LConn1

== system T6_changeloadmodeltocurrentload_v1/Wind energy/Subsystem1 ==
  In1 : Inport
  Square1 : Math  Operator=pow
  power of 3 : Constant  Value=3
  Out1 : Outport
  wires:
  power of 3/1 -> Square1/2
  Square1/1 -> Out1/1
  In1/1 -> Square1/1

== matlab function T6_changeloadmodeltocurrentload_v1/Subsystem/MATLAB Function ==
  data: button1 input; button2 input; button3 input; button4 input; data1 input; data2 input; y output; data3 input; data4 input
function y = fcn(button1, button2, button3, button4, data1,data2,data3, data4)
    if button1
        y = data1;
    elseif button2
        y =data2;
    elseif button3
        y = data3;
    elseif button4
        y = data4;
    else 
        y = data1;
    end
end

== matlab function T6_changeloadmodeltocurrentload_v1/Solar power/MPPT/MPPT Controller using Perturb & Observe technique  ==
  settings: updateMethod=DISCRETE  sampleTime=0.01
  data: Param input; Enabled input; V input; I input; D output
function D  = PandO(Param, Enabled, V, I)

% MPPT controller based on the Perturb & Observe algorithm.

% D output = Duty cycle of the boost converter (value between 0 and 1)
%
% Enabled input = 1 to enable the MPPT controller
% V input = PV array terminal voltage (V)
% I input = PV array current (A)
%
% Param input:
Dinit = Param(1);  %Initial value for D output
Dmax = Param(2);   %Maximum value for D
Dmin = Param(3);   %Minimum value for D
deltaD = Param(4); %Increment value used to increase/decrease the duty cycle D
% ( increasing D = decreasing Vref )
%  

persistent Vold Pold Dold;

dataType = 'double';

if isempty(Vold)
    Vold=0;
    Pold=0;
    Dold=Dinit;
end
P= V*I;
dV= V - Vold;
dP= P - Pold;

 if dP ~= 0 & Enabled ~=0
%     if dP>1e-9  & dP<-1e-9 & Enabled ~=0
    if dP < 0
        if dV < 0
            D = Dold - deltaD;
        else
            D = Dold + deltaD;
        end
    else
        if dV < 0
            D = Dold + deltaD;
        else
            D = Dold - deltaD;
        end    
    end
else D=Dold;
end

if D >= Dmax | D<= Dmin
    D=Dold;
end

Dold=D;
Vold=V;
Pold=P;

== stateflow chart T6_changeloadmodeltocurrentload_v1/Chart ==
  settings: executeAtInitialization=1
  state Button1selected
  state Button2selected
  state Button3selected
  state Button4selected
  Button1selected -> Button4selected [order 4] : [Button4pressed]
  Button2selected -> Button4selected [order 4] : [Button4pressed]
  Button1selected -> Button3selected [order 3] : [Button3pressed]
  (default) -> Button1selected
  Button3selected -> Button4selected [order 2] : [Button4pressed]
  Button2selected -> Button3selected [order 2] : [Button3pressed]
  Button1selected -> Button1selected [order 2] : [Button1pressed]
  Button3selected -> Button2selected [order 1] : [Button2pressed]
  Button4selected -> Button4selected [order 2] : [Button4pressed]
  Button1selected -> Button2selected [order 1] : [Button2pressed]
  Button4selected -> Button3selected [order 1] : [Button3pressed]
  Button2selected -> Button1selected [order 1] : [Button1pressed]
  Button3selected -> Button3selected [order 3] : [Button3pressed]
  Button3selected -> Button1selected [order 4] : [Button1pressed]
  Button4selected -> Button1selected [order 3] : [Button1pressed]
  Button2selected -> Button2selected [order 3] : [Button2pressed]
  Button4selected -> Button2selected [order 4] : [Button2pressed]
  data: Button1selected output boolean; Button2selected output boolean; Button3selected output boolean; Button1pressed input boolean size=1; Button2pressed input boolean size=1; Button3pressed input boolean size=1; Button4pressed input boolean size=1; Button4selected output boolean

== matlab function T6_changeloadmodeltocurrentload_v1/Household1/MATLAB Function ==
  data: button1 input; button2 input; button3 input; button4 input; data1 input; data2 input; y output; data3 input; data4 input
function y = fcn(button1, button2, button3, button4, data1,data2,data3, data4)
    if button1
        y = data1;
    elseif button2
        y =data2;
    elseif button3
        y = data3;
    elseif button4
        y = data4;
    else 
        y = data1;
    end
end

== matlab function T6_changeloadmodeltocurrentload_v1/Household2/MATLAB Function ==
  data: button1 input; button2 input; button3 input; button4 input; data1 input; data2 input; y output; data3 input; data4 input
function y = fcn(button1, button2, button3, button4, data1,data2,data3, data4)
    if button1
        y = data1;
    elseif button2
        y =data2;
    elseif button3
        y = data3;
    elseif button4
        y = data4;
    else 
        y = data1;
    end
end

== matlab function T6_changeloadmodeltocurrentload_v1/Household3/MATLAB Function ==
  data: button1 input; button2 input; button3 input; button4 input; data1 input; data2 input; y output; data3 input; data4 input
function y = fcn(button1, button2, button3, button4, data1,data2,data3, data4)
    if button1
        y = data1;
    elseif button2
        y =data2;
    elseif button3
        y = data3;
    elseif button4
        y = data4;
    else 
        y = data1;
    end
end

== matlab function T6_changeloadmodeltocurrentload_v1/Household4/MATLAB Function ==
  data: button1 input; button2 input; button3 input; button4 input; data1 input; data2 input; y output; data3 input; data4 input
function y = fcn(button1, button2, button3, button4, data1,data2,data3, data4)
    if button1
        y = data1;
    elseif button2
        y =data2;
    elseif button3
        y = data3;
    elseif button4
        y = data4;
    else 
        y = data1;
    end
end

== matlab function T6_changeloadmodeltocurrentload_v1/Household5/MATLAB Function ==
  data: button1 input; button2 input; button3 input; button4 input; data1 input; data2 input; y output; data3 input; data4 input
function y = fcn(button1, button2, button3, button4, data1,data2,data3, data4)
    if button1
        y = data1;
    elseif button2
        y =data2;
    elseif button3
        y = data3;
    elseif button4
        y = data4;
    else 
        y = data1;
    end
end

== matlab function T6_changeloadmodeltocurrentload_v1/Household6/MATLAB Function ==
  data: button1 input; button2 input; button3 input; button4 input; data1 input; data2 input; y output; data3 input; data4 input
function y = fcn(button1, button2, button3, button4, data1,data2,data3, data4)
    if button1
        y = data1;
    elseif button2
        y =data2;
    elseif button3
        y = data3;
    elseif button4
        y = data4;
    else 
        y = data1;
    end
end

== matlab function T6_changeloadmodeltocurrentload_v1/Household7/MATLAB Function ==
  data: button1 input; button2 input; button3 input; button4 input; data1 input; data2 input; y output; data3 input; data4 input
function y = fcn(button1, button2, button3, button4, data1,data2,data3, data4)
    if button1
        y = data1;
    elseif button2
        y =data2;
    elseif button3
        y = data3;
    elseif button4
        y = data4;
    else 
        y = data1;
    end
end

== matlab function T6_changeloadmodeltocurrentload_v1/Household8/MATLAB Function ==
  data: button1 input; button2 input; button3 input; button4 input; data1 input; data2 input; y output; data3 input; data4 input
function y = fcn(button1, button2, button3, button4, data1,data2,data3, data4)
    if button1
        y = data1;
    elseif button2
        y =data2;
    elseif button3
        y = data3;
    elseif button4
        y = data4;
    else 
        y = data1;
    end
end

== matlab function T6_changeloadmodeltocurrentload_v1/Household9/MATLAB Function ==
  data: button1 input; button2 input; button3 input; button4 input; data1 input; data2 input; y output; data3 input; data4 input
function y = fcn(button1, button2, button3, button4, data1,data2,data3, data4)
    if button1
        y = data1;
    elseif button2
        y =data2;
    elseif button3
        y = data3;
    elseif button4
        y = data4;
    else 
        y = data1;
    end
end

== matlab function T6_changeloadmodeltocurrentload_v1/Household11/MATLAB Function ==
  data: button1 input; button2 input; button3 input; button4 input; data1 input; data2 input; y output; data3 input; data4 input
function y = fcn(button1, button2, button3, button4, data1,data2,data3, data4)
    if button1
        y = data1;
    elseif button2
        y =data2;
    elseif button3
        y = data3;
    elseif button4
        y = data4;
    else 
        y = data1;
    end
end

== matlab function T6_changeloadmodeltocurrentload_v1/Household12/MATLAB Function ==
  data: button1 input; button2 input; button3 input; button4 input; data1 input; data2 input; y output; data3 input; data4 input
function y = fcn(button1, button2, button3, button4, data1,data2,data3, data4)
    if button1
        y = data1;
    elseif button2
        y =data2;
    elseif button3
        y = data3;
    elseif button4
        y = data4;
    else 
        y = data1;
    end
end

== matlab function T6_changeloadmodeltocurrentload_v1/Household13/MATLAB Function ==
  data: button1 input; button2 input; button3 input; button4 input; data1 input; data2 input; y output; data3 input; data4 input
function y = fcn(button1, button2, button3, button4, data1,data2,data3, data4)
    if button1
        y = data1;
    elseif button2
        y =data2;
    elseif button3
        y = data3;
    elseif button4
        y = data4;
    else 
        y = data1;
    end
end

== matlab function T6_changeloadmodeltocurrentload_v1/Subsystem1/MATLAB Function ==
  data: button1 input; button2 input; button3 input; button4 input; data1 input; data2 input; y output; data3 input; data4 input
function y = fcn(button1, button2, button3, button4, data1,data2,data3, data4)
    if button1
        y = data1;
    elseif button2
        y =data2;
    elseif button3
        y = data3;
    elseif button4
        y = data4;
    else 
        y = data1;
    end
end

== matlab function T6_changeloadmodeltocurrentload_v1/Household10/MATLAB Function ==
  data: button1 input; button2 input; button3 input; button4 input; data1 input; data2 input; y output; data3 input; data4 input
function y = fcn(button1, button2, button3, button4, data1,data2,data3, data4)
    if button1
        y = data1;
    elseif button2
        y =data2;
    elseif button3
        y = data3;
    elseif button4
        y = data4;
    else 
        y = data1;
    end
end
